simulink model "chap6_3sim"  (Simulink 7.7)
settings: Solver=ode45  StartTime=0.0  StopTime=10  RelTol=1e-3
settings Model: Creator=ljk  LastModifiedBy=ljk  ExtModeTrigMode=oneshot  ExtModeArmWhenConnect=off
settings DataIOCC: LimitDataPoints=off
settings OptimizationCC: BlockReduction=off  BooleanDataType=off
settings DebuggingCC: SaveWithParameterizedLinksMsg=none  SignalResolutionControl=TryResolveAllWithWarning  SolverPrmCheckMsg=none  MultiTaskDSMMsg=warning  MultiTaskCondExecSysMsg=none  StrictBusMsg=None
settings HardwareCC: TargetUnknown=on
settings RTWCC: IncludeERTFirstTime=on

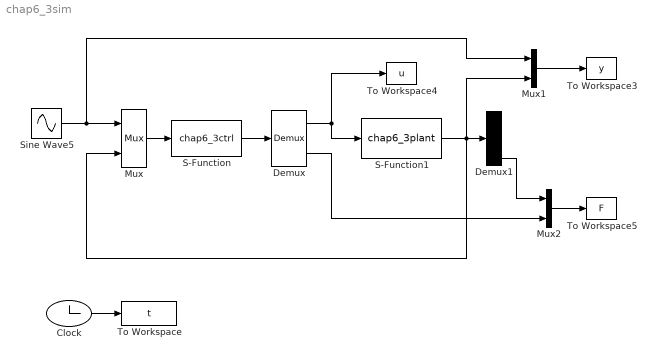
== system chap6_3sim ==
  Clock : Clock
  Demux : Demux  Outputs=2
  Demux1 : Demux  Outputs=3
  Mux : Mux  Inputs=2
  Mux1 : Mux  Inputs=2
  Mux2 : Mux  Inputs=2
  S-Function : S-Function  FunctionName=chap6_3ctrl  EnableBusSupport=off
  S-Function1 : S-Function  FunctionName=chap6_3plant  EnableBusSupport=off
  Sine Wave5 : Sin  SampleTime=0
  To Workspace : ToWorkspace  VariableName=t  SampleTime=-1  SaveFormat=Array
  To Workspace3 : ToWorkspace  VariableName=y  SampleTime=-1  SaveFormat=Array
  To Workspace4 : ToWorkspace  VariableName=u  SampleTime=-1  SaveFormat=Array
  To Workspace5 : ToWorkspace  VariableName=F  SampleTime=-1  SaveFormat=Array
  wires:
  Mux/1 -> S-Function/1
  S-Function1/1 -> Mux/2, Demux1/1, Mux1/2
  S-Function/1 -> Demux/1
  Demux/1 -> S-Function1/1, To Workspace4/1
  Sine Wave5/1 -> Mux/1, Mux1/1
  Mux1/1 -> To Workspace3/1
  Clock/1 -> To Workspace/1
  Mux2/1 -> To Workspace5/1
  Demux1/3 -> Mux2/1
  Demux/2 -> Mux2/2
